simulink model "e2a"  (R2021a)
settings: Solver=VariableStepAuto  StartTime=0.0  StopTime=10.0  RelTol=1e-3
libraries: visionsources x1
settings Model: Creator=pranshu  LastModifiedBy=pranshu

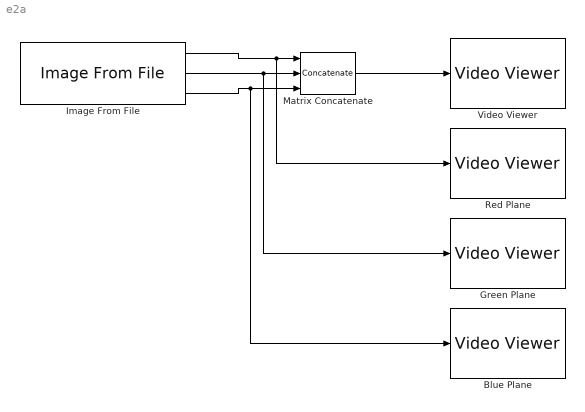
== system e2a ==
  Blue Plane : VideoViewer  FigPos=[559 583 418 304]
  Green Plane : VideoViewer  FigPos=[559 583 418 304]
  Image From File : visionsources/Image From File  Tag=vipblks_nd  FileName=peppers.png  Ts=inf  imagePorts=Separate color signals  OutPortLabels=R|G|B  ImageDataType=Inherit from input image  sdImageDataType=uint(8)  Signed=on  WordLength=16  FractionLengthMode=User-defined  FractionLength=15
  Matrix Concatenate : Concatenate  NumInputs=3  Mode=Multidimensional array  ConcatenateDimension=3
  Red Plane : VideoViewer  FigPos=[559 583 418 304]
  Video Viewer : VideoViewer  FigPos=[121.8 579.6 417.6 304]
  wires:
  Matrix Concatenate/1 -> Video Viewer/1
  Image From File/2 -> Green Plane/1, Matrix Concatenate/2
  Image From File/1 -> Red Plane/1, Matrix Concatenate/1
  Image From File/3 -> Blue Plane/1, Matrix Concatenate/3
